simulink model "new_overtaking_085_mp"  (Simulink 10.2)
settings: Solver=VariableStepAuto  StartTime=0.0  StopTime=45  RelTol=1e-3
libraries: Solver_SF x1
settings Model: Creator=陈莹  LastModifiedBy=26952
settings SolverCC: AlgebraicLoopSolver=LineSearch
settings DataIOCC: SaveFormat=Dataset  SignalLoggingSaveFormat=Dataset
settings OptimizationCC: LifeSpan=auto
settings DebuggingCC: UnderspecifiedInitializationDetection=Simplified  MergeDetectMultiDrivingBlocksExec=error  FcnCallInpInsideContextMsg=error  SFUnexpectedBacktrackingDiag=error  SFNoUnconditionalDefaultTransitionDiag=error  SFExecutionAtInitializationDiag=warning
settings HardwareCC: ProdBitPerPointer=64  ProdBitPerSizeT=64  ProdBitPerPtrDiffT=64  ProdLargestAtomicFloat=Float  ProdIntDivRoundTo=Zero  ProdEndianess=LittleEndian  ProdWordSize=64  ProdHWDeviceType=Intel->x86-64 (Windows64)
settings ModelReferenceCC: PropagateSignalLabelsOutOfModel=on
settings SFSimCC: SimUseLocalCustomCode=on
settings RTWCC: RTWUseLocalCustomCode=on
settings CodeAppCC: StateflowObjectComments=off
settings GRTTargetCC: TargetLangStandard=C99 (ISO)  CombineOutputUpdateFcns=on  GRTInterface=off
settings ConfigComp: CovMetricSettings=dwe  CovSaveCumulativeToWorkspaceVar=off  CovSaveSingleToWorkspaceVar=off  CovExternalEMLEnable=on

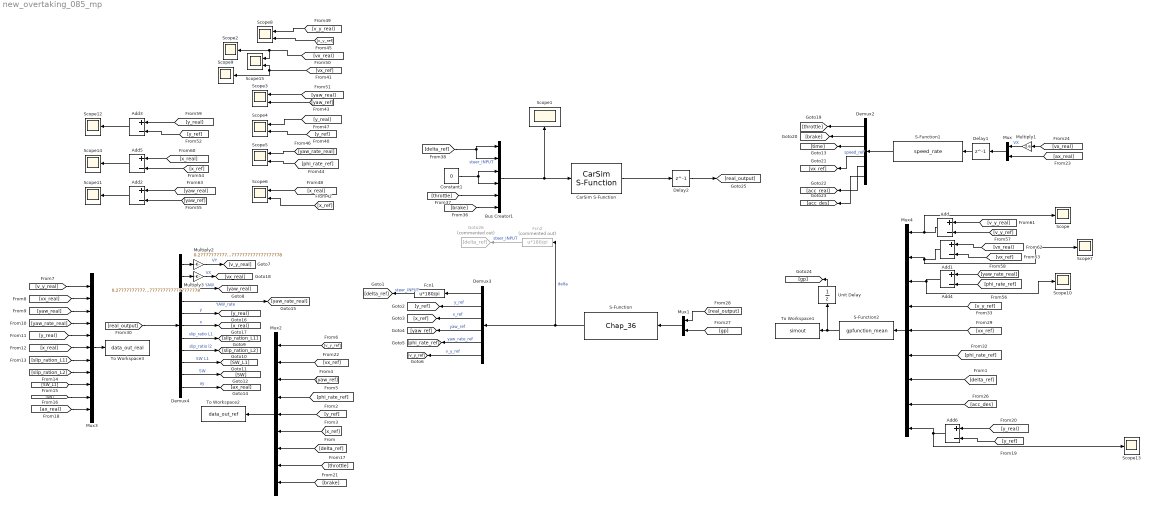
== system new_overtaking_085_mp ==
  Add{,1..6} (7 alike) : Sum  Inputs=+-
  Bus Creator1 : BusCreator  Inputs=6
  CarSim S-Function : Solver_SF/CarSim S-Function  Priority=1  SIMFILE=simfile.sim
  Constant1 : Constant  Value=0
  Delay1 : Delay  DelayLength=1  InitialCondition=0
  Delay2 : Delay  DelayLength=1  InitialCondition=0
  Demux2 : Demux  Outputs=6
  Demux3 : Demux  Outputs=6
  Demux4 : Demux  Outputs=11
  Fcn1 : Fcn  Expr=u*180/pi
  Fcn2 : Fcn  Commented=on  Expr=u*180/pi
  Goto26 : Goto  Commented=on  GotoTag=delta_ref
  Multiply1 : Gain  Gain=3.6
  Multiply2 : Gain  Gain=0.27777777777777777777777777777778
  Multiply3 : Gain  Gain=0.27777777777777777777777777777778
  Mux : Mux  Inputs=2
  Mux1 : Mux  Inputs=2
  Mux2 : Mux  Inputs=9
  Mux3 : Mux  Inputs=11
  Mux4 : Mux  Inputs=9
  S-Function : S-Function  FunctionName=Chap_36  SFunctionDeploymentMode=off  EnableBusSupport=off
  S-Function1 : S-Function  FunctionName=speed_rate  SFunctionDeploymentMode=off  EnableBusSupport=off
  S-Function2 : S-Function  FunctionName=gpfunction_mean  SFunctionDeploymentMode=off  EnableBusSupport=off
  Scope{,1..2,7,9..14} (10 alike) : Scope
  Scope{3..6,8,15} (6 alike) : Scope  NumInputPorts=2
  To Workspace1 : ToWorkspace  VariableName=simout  SaveFormat=Timeseries  SampleTime=-1
  To Workspace2 : ToWorkspace  VariableName=data_out_ref  SaveFormat=Timeseries  SampleTime=-1
  To Workspace3 : ToWorkspace  VariableName=data_out_real  SaveFormat=Timeseries  SampleTime=-1
  Unit Delay : UnitDelay  SampleTime=-1  HasFrameUpgradeWarning=on
  wires:
  S-Function/1 -> Fcn2/1, Demux3/1  "delta"
  CarSim S-Function/1 -> Delay2/1
  Delay2/1 -> [real_output]
  Bus Creator1/1 -> CarSim S-Function/1, Scope1/1
  Demux3/1 -> Fcn1/1
  Demux4/1 -> Multiply2/1
  Demux4/2 -> Multiply3/1
  Mux4/1 -> S-Function2/1
  S-Function2/1 -> Unit Delay/1, To Workspace1/1
  Multiply2/1 -> [v_y_real]  "VY"
  Multiply3/1 -> [vx_real]  "VX"
  Demux4/3 -> [yaw_real]  "YAW"
  Demux4/4 -> [yaw_rate_real]  "YAW_rate"
  Demux4/5 -> [y_real]  "y"
  Demux4/6 -> [x_real]  "x"
  Demux4/7 -> [slip_ration_L1]  "slip_ratio L1"
  Demux4/8 -> [slip_ration_L2]  "slip_ratio l2"
  Demux4/9 -> [SW_L1]  "SW L1"
  Demux4/10 -> [SW]  "SW"
  Demux4/11 -> [ax_real]  "ay"
  Demux3/6 -> [v_y_ref]  "v_y_ref"
  Demux3/2 -> [y_ref]  "y_ref"
  Demux3/4 -> [yaw_ref]  "yaw_ref"
  Demux3/5 -> [phi_rate_ref]  "yaw_rate_ref"
  Demux3/3 -> [x_ref]  "x_ref"
  Fcn1/1 -> [delta_ref]  "steer_INPUT"
  [x_ref] -> Scope6/2
  [y_ref] -> Scope4/2
  [yaw_ref] -> Scope3/2
  [vx_ref] -> Scope15/2, Scope9/1
  [v_y_ref] -> Scope8/2
  [vx_real] -> Scope15/1, Scope2/1
  [yaw_real] -> Scope3/1
  [y_real] -> Scope4/1
  [yaw_rate_real] -> Scope5/1
  [phi_rate_ref] -> Scope5/2
  [x_real] -> Scope6/1
  [ax_real] -> Mux/2
  Demux2/3 -> [time]
  Demux2/6 -> [acc_des]
  Demux2/1 -> [throttle]
  Demux2/5 -> [acc_real]
  Delay1/1 -> S-Function1/1
  [vx_real] -> Multiply1/1
  Mux/1 -> Delay1/1
  S-Function1/1 -> Demux2/1
  Multiply1/1 -> Mux/1  "VX"
  Demux2/4 -> [vx_ref]  "speed_ref"
  Demux2/2 -> [brake]
  [throttle] -> Mux2/8
  [SW] -> Mux3/10
  [y_ref] -> Mux2/5
  [x_ref] -> Mux2/6
  [y_real] -> Mux3/5
  [yaw_real] -> Mux3/3
  [yaw_ref] -> Mux2/3
  [SW_L1] -> Mux3/9
  [brake] -> Mux2/9
  [ax_real] -> Mux3/11
  [phi_rate_ref] -> Mux2/4
  Mux2/1 -> To Workspace2/1
  [v_y_ref] -> Mux2/1
  [slip_ration_L2] -> Mux3/8
  [delta_ref] -> Mux2/7
  [v_y_real] -> Mux3/1
  [yaw_rate_real] -> Mux3/4
  [vx_ref] -> Mux2/2
  [slip_ration_L1] -> Mux3/7
  [vx_real] -> Mux3/2
  [x_real] -> Mux3/6
  Mux3/1 -> To Workspace3/1
  [v_y_real] -> Scope8/1
  [v_y_real] -> Add/1
  [v_y_ref] -> Add/2
  [vx_real] -> Add1/1
  [vx_ref] -> Add1/2
  [yaw_real] -> Add2/1
  [yaw_ref] -> Add2/2
  [y_real] -> Add3/1
  [y_ref] -> Add3/2
  [yaw_rate_real] -> Add4/1
  [phi_rate_ref] -> Add4/2
  [x_ref] -> Add5/2
  [x_real] -> Add5/1
  Add/1 -> Scope/1, Mux4/1
  Add1/1 -> Scope7/1, Mux4/2
  Add2/1 -> Scope11/1
  Add3/1 -> Scope12/1
  Add4/1 -> Scope10/1, Mux4/3
  Add5/1 -> Scope14/1
  [v_y_ref] -> Mux4/4
  [vx_ref] -> Mux4/5
  [phi_rate_ref] -> Mux4/6
  [delta_ref] -> Mux4/7
  [acc_des] -> Mux4/8
  [real_output] -> Demux4/1
  [real_output] -> Mux1/1
  [gp] -> Mux1/2
  Unit Delay/1 -> [gp]
  Constant1/1 -> Bus Creator1/4, Bus Creator1/3
  [brake] -> Bus Creator1/6
  [throttle] -> Bus Creator1/5
  [delta_ref] -> Bus Creator1/1, Bus Creator1/2  "steer_INPUT"
  Fcn2/1 -> Goto26/1  "steer_INPUT"
  Add6/1 -> Mux4/9, Scope13/1
  [y_real] -> Add6/1
  [y_ref] -> Add6/2
  Mux1/1 -> S-Function/1
